simulink model "Quadcopter_simLINEAR"  (R2021a)
settings: Solver=VariableStepAuto  StartTime=0.0  StopTime=t_stop  RelTol=1e-3
values from neighbouring files (symbols this model uses):
  b = 0.001    [Exercise2.m]    (also in Exercise2_3.m)
  Dx = 0.01    [Exercise2.m]    (also in Exercise2_3.m)
  Dy = 0.01    [Exercise2.m]    (also in Exercise2_3.m)
  Dz = 0.01    [Exercise2.m]    (also in Exercise2_3.m)
  g = 9.81    [Exercise2.m]    (also in Exercise2_3.m)
  Ixx = 3e-06    [Exercise2.m]    (also in Exercise2_3.m)
  Iyy = 3e-06    [Exercise2.m]    (also in Exercise2_3.m)
  Izz = 1e-05    [Exercise2.m]    (also in Exercise2_3.m)
  k = 0.01    [Exercise2.m]    (also in Exercise2_3.m)
  L = 0.225    [Exercise2.m]    (also in Exercise2_3.m)
  m = 0.5    [Exercise2.m]    (also in Exercise2_3.m)
  omega1 = 10000    [Exercise2_3.m]
  omega2 = 0    [Exercise2_3.m]
  omega3 = 10000    [Exercise2_3.m]
  omega4 = 0    [Exercise2_3.m]
libraries: vrlib x1
settings Model: Creator=emilm  LastModifiedBy=emilm

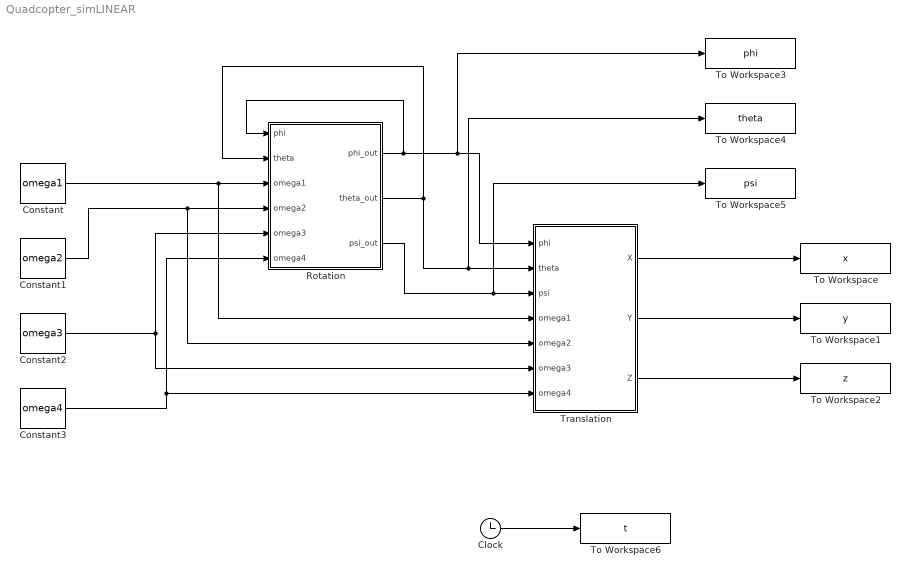
== system Quadcopter_simLINEAR ==
  Clock : Clock
  Constant : Constant  Value=omega1
  Constant1 : Constant  Value=omega2
  Constant2 : Constant  Value=omega3
  Constant3 : Constant  Value=omega4
  Rotation : Subsystem
  To Workspace : ToWorkspace  VariableName=x  SampleTime=-1
  To Workspace1 : ToWorkspace  VariableName=y  SampleTime=-1
  To Workspace2 : ToWorkspace  VariableName=z  SampleTime=-1
  To Workspace3 : ToWorkspace  VariableName=phi  SampleTime=-1
  To Workspace4 : ToWorkspace  VariableName=theta  SampleTime=-1
  To Workspace5 : ToWorkspace  VariableName=psi  SampleTime=-1
  To Workspace6 : ToWorkspace  VariableName=t  SampleTime=-1
  Translation : Subsystem
  wires:
  Rotation/1(phi_out) -> Rotation/1(phi), To Workspace3/1, Translation/1(phi)
  Rotation/2(theta_out) -> To Workspace4/1, Translation/2(theta), Rotation/2(theta)
  Rotation/3(psi_out) -> To Workspace5/1, Translation/3(psi)
  Constant/1 -> Translation/4(omega1), Rotation/3(omega1)
  Constant1/1 -> Translation/5(omega2), Rotation/4(omega2)
  Constant2/1 -> Rotation/5(omega3), Translation/6(omega3)
  Constant3/1 -> Translation/7(omega4), Rotation/6(omega4)
  Translation/1(X) -> To Workspace/1
  Translation/2(Y) -> To Workspace1/1
  Translation/3(Z) -> To Workspace2/1
  Clock/1 -> To Workspace6/1

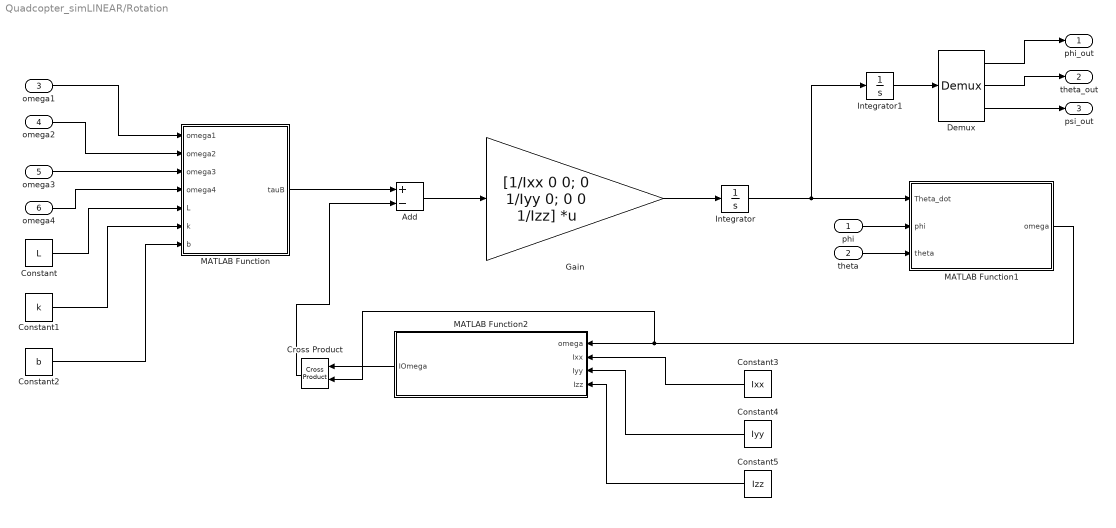
== system Quadcopter_simLINEAR/Rotation ==
  phi : Inport
  theta : Inport  Port=2
  omega1 : Inport  Port=3
  omega2 : Inport  Port=4
  omega3 : Inport  Port=5
  omega4 : Inport  Port=6
  Add : Sum  Inputs=+-
  Constant : Constant  Value=L
  Constant1 : Constant  Value=k
  Constant2 : Constant  Value=b
  Constant3 : Constant  Value=Ixx
  Constant4 : Constant  Value=Iyy
  Constant5 : Constant  Value=Izz
  Cross Product : vrlib/Utilities/Cross Product
  Demux : Demux  Outputs=3
  Gain : Gain  Gain=[1/Ixx 0 0; 0 1/Iyy 0; 0 0 1/Izz]  Multiplication=Matrix(K*u)
  Integrator : Integrator
  Integrator1 : Integrator
  MATLAB Function : MATLAB Function  TreatAsAtomicUnit=on
  MATLAB Function1 : MATLAB Function  TreatAsAtomicUnit=on
  MATLAB Function2 : MATLAB Function  TreatAsAtomicUnit=on
  phi_out : Outport
  theta_out : Outport  Port=2
  psi_out : Outport  Port=3
  wires:
  omega1/1 -> MATLAB Function/1(omega1)
  omega2/1 -> MATLAB Function/2(omega2)
  omega3/1 -> MATLAB Function/3(omega3)
  omega4/1 -> MATLAB Function/4(omega4)
  Constant/1 -> MATLAB Function/5(L)
  Constant1/1 -> MATLAB Function/6(k)
  Constant2/1 -> MATLAB Function/7(b)
  MATLAB Function/1(tauB) -> Add/1
  Add/1 -> Gain/1
  Gain/1 -> Integrator/1
  Integrator/1 -> Integrator1/1, MATLAB Function1/1(Theta_dot)
  phi/1 -> MATLAB Function1/2(phi)
  theta/1 -> MATLAB Function1/3(theta)
  MATLAB Function1/1(omega) -> Cross Product/2, MATLAB Function2/1(omega)
  Integrator1/1 -> Demux/1
  Demux/1 -> phi_out/1
  Demux/2 -> theta_out/1
  Demux/3 -> psi_out/1
  Constant3/1 -> MATLAB Function2/2(Ixx)
  Constant4/1 -> MATLAB Function2/3(Iyy)
  Constant5/1 -> MATLAB Function2/4(Izz)
  MATLAB Function2/1(IOmega) -> Cross Product/1
  Cross Product/1 -> Add/2

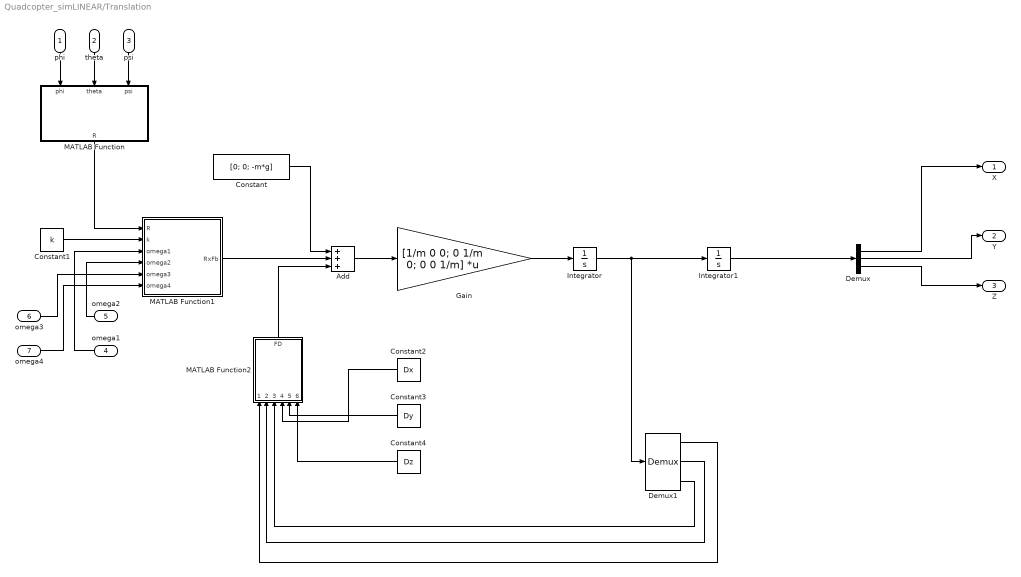
== system Quadcopter_simLINEAR/Translation ==
  phi : Inport
  theta : Inport  Port=2
  psi : Inport  Port=3
  omega1 : Inport  Port=4
  omega2 : Inport  Port=5
  omega3 : Inport  Port=6
  omega4 : Inport  Port=7
  Add : Sum  Inputs=+++
  Constant : Constant  Value=[0; 0; -m*g]
  Constant1 : Constant  Value=k
  Constant2 : Constant  Value=Dx
  Constant3 : Constant  Value=Dy
  Constant4 : Constant  Value=Dz
  Demux : Demux  Outputs=3
  Demux1 : Demux  Outputs=3
  Gain : Gain  Gain=[1/m 0 0; 0 1/m 0; 0 0 1/m]  Multiplication=Matrix(K*u)
  Integrator : Integrator
  Integrator1 : Integrator
  MATLAB Function : MATLAB Function  TreatAsAtomicUnit=on
  MATLAB Function1 : MATLAB Function  TreatAsAtomicUnit=on
  MATLAB Function2 : MATLAB Function  TreatAsAtomicUnit=on
  X : Outport
  Y : Outport  Port=2
  Z : Outport  Port=3
  wires:
  Gain/1 -> Integrator/1
  theta/1 -> MATLAB Function/2(theta)
  psi/1 -> MATLAB Function/3(psi)
  phi/1 -> MATLAB Function/1(phi)
  Add/1 -> Gain/1
  Constant/1 -> Add/1
  MATLAB Function1/1(RxFb) -> Add/2
  MATLAB Function/1(R) -> MATLAB Function1/1(R)
  Constant1/1 -> MATLAB Function1/2(k)
  omega2/1 -> MATLAB Function1/4(omega2)
  omega1/1 -> MATLAB Function1/3(omega1)
  omega3/1 -> MATLAB Function1/5(omega3)
  omega4/1 -> MATLAB Function1/6(omega4)
  Integrator/1 -> Demux1/1, Integrator1/1
  Integrator1/1 -> Demux/1
  Demux/1 -> X/1
  Demux/2 -> Y/1
  Demux/3 -> Z/1
  MATLAB Function2/1(FD) -> Add/3
  Constant2/1 -> MATLAB Function2/4(Dx)
  Constant3/1 -> MATLAB Function2/5(Dy)
  Constant4/1 -> MATLAB Function2/6(Dz)
  Demux1/1 -> MATLAB Function2/1(x_dot)
  Demux1/2 -> MATLAB Function2/2(y_dot)
  Demux1/3 -> MATLAB Function2/3(z_dot)

== matlab function Quadcopter_simLINEAR/Translation/MATLAB Function1 ==
  data: R input; RxFb output; k input; omega1 input; omega2 input; omega3 input; omega4 input
function RxFb = RxFb(R, k, omega1, omega2, omega3, omega4)

RxFb = R*[0; 0; k*(omega1^2+omega2^2+omega3^2+omega4^2)];

== matlab function Quadcopter_simLINEAR/Translation/MATLAB Function ==
  data: phi input; R output; theta input; psi input
function R = R(phi, theta, psi)

% c1 = cos(phi);
% c2 = cos(theta);
% c3 = cos(psi);
% 
% s1 = sin(phi);
% s2 = sin(theta);
% s3 = sin(psi);


% R = [c3*c2 c3*s2*s1-s3*c1 c3*s2*c1+s3*s1;
%      s3*c2 s3*s2*s1+c3*c1 s3*s2*c1-c3*s1
%      -s2         c2*s1        c2*c1];
R = [1 theta*phi-psi theta+psi*phi;
    psi psi*theta*phi+1 psi*theta-phi;
    -theta phi 1];

== matlab function Quadcopter_simLINEAR/Translation/MATLAB Function2 ==
  data: x_dot input; y_dot input; z_dot input; FD output; Dx input; Dy input; Dz input
function FD = FD(x_dot, y_dot, z_dot, Dx, Dy, Dz)

D = [Dx 0 0; 0 Dy 0; 0 0 Dz];

FD = D*[x_dot; y_dot; z_dot];

== matlab function Quadcopter_simLINEAR/Rotation/MATLAB Function ==
  data: omega1 input; tauB output; omega2 input; omega3 input; omega4 input; L input; k input; b input
function tauB = tauB(omega1, omega2, omega3, omega4, L, k, b)

tauB = [L*k*(omega1^2-omega3^2);
        L*k*(omega2^2-omega4^2);
        b*(omega1^2-omega2^2+omega3^2-omega4^2)];

== matlab function Quadcopter_simLINEAR/Rotation/MATLAB Function1 ==
  data: Theta_dot input; omega output; phi input; theta input
function omega = omega(Theta_dot, phi, theta)

% R = [1 0 -sin(theta);
%      0 cos(phi) cos(theta)*sin(phi);
%      0 -sin(phi) cos(theta)*cos(phi)];

R = [1 0 -theta;
    0 1 phi;
    0 -phi 1];
 
 omega = R*Theta_dot;

== matlab function Quadcopter_simLINEAR/Rotation/MATLAB Function2 ==
  data: omega input; IOmega output; Ixx input; Iyy input; Izz input
function IOmega = Iomega(omega, Ixx, Iyy, Izz)



IOmega = [Ixx 0 0; 0 Iyy 0; 0 0 Izz]*omega;
